simulink model "Controls"  (R2020b)
settings: Solver=VariableStepAuto  StartTime=0.0  StopTime=10.0  RelTol=1e-3
settings Model: Creator=macra  LastModifiedBy=macra

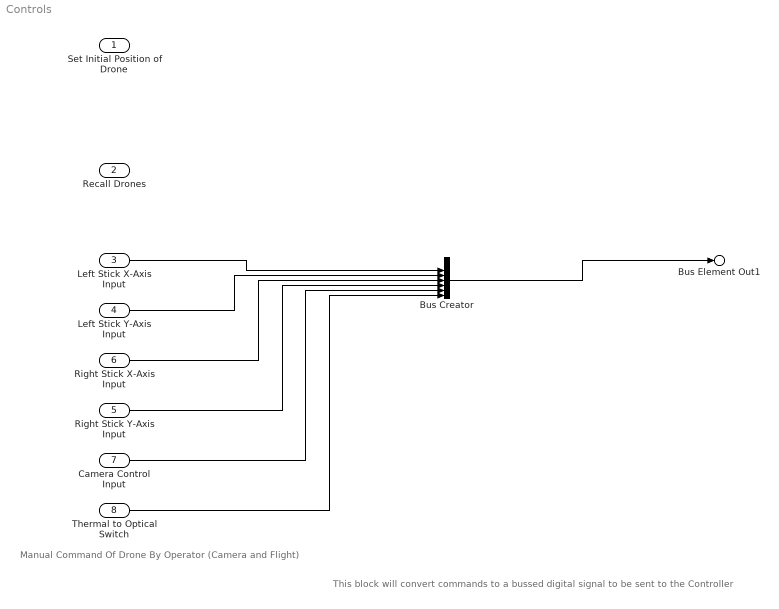
== system Controls ==
  note: This block will convert commands to a bussed digital signal to be sent to the Controller
  note: Manual Command Of Drone By Operator (Camera and Flight)
  Set Initial Position of Drone : Inport
  Recall Drones : Inport  Port=2
  Left Stick X-Axis Input : Inport  Port=3
  Left Stick Y-Axis Input : Inport  Port=4
  Right Stick Y-Axis Input : Inport  Port=5
  Right Stick X-Axis Input : Inport  Port=6
  Camera Control Input : Inport  Port=7
  Thermal to Optical Switch : Inport  Port=8
  Bus Creator : BusCreator  Inputs=8
  Bus Element Out1 : Outport  PortName=Input Commands
  wires:
  Bus Creator/1 -> Bus Element Out1/1
  Left Stick X-Axis Input/1 -> Bus Creator/3
  Left Stick Y-Axis Input/1 -> Bus Creator/4
  Right Stick X-Axis Input/1 -> Bus Creator/5
  Right Stick Y-Axis Input/1 -> Bus Creator/6
  Camera Control Input/1 -> Bus Creator/7
  Thermal to Optical Switch/1 -> Bus Creator/8
